simulink model "Quaternions"  (R2021b)
settings: Solver=VariableStepAuto  StartTime=0.0  StopTime=SimTime  MaxStep=1e-2  RelTol=1e-13
values from neighbouring files (symbols this model uses):
  q0 = [0 0 1 0]    [Lab_4.m]
libraries: robotcorelib x1, vrlib x1
settings Model: Creator=adity  LastModifiedBy=adity
settings SolverCC: AlgebraicLoopSolver=TrustRegion
settings DebuggingCC: SFMachineParentedDataDiag=warning

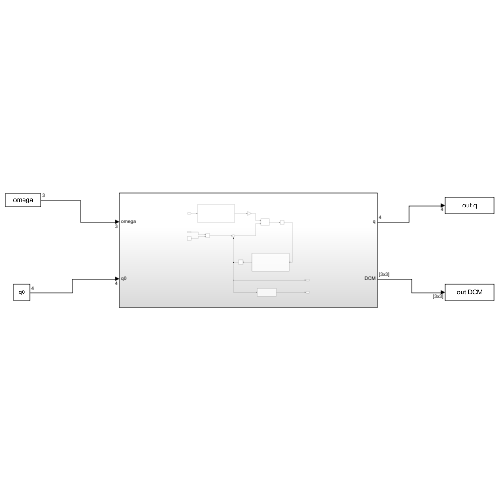
[thumbnail: Simulink's stored preview of the top-level diagram]
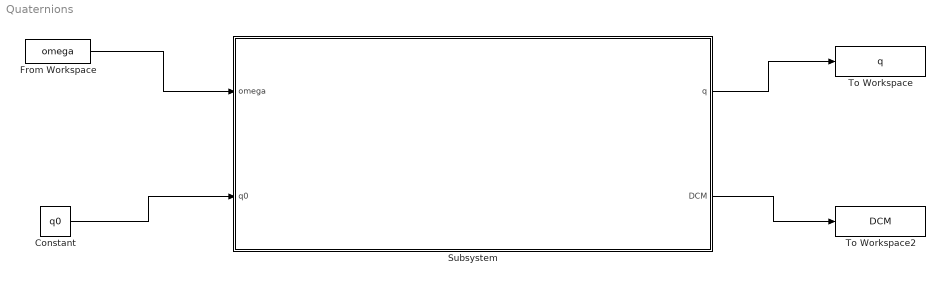
== system Quaternions ==
  Constant : Constant  Value=q0
  From Workspace : FromWorkspace  VariableName=omega
  Subsystem : Subsystem
  To Workspace : ToWorkspace  VariableName=q  SaveFormat=Timeseries  SampleTime=-1
  To Workspace2 : ToWorkspace  VariableName=DCM  SaveFormat=Timeseries  SampleTime=-1
  wires:
  From Workspace/1 -> Subsystem/1(omega)
  Constant/1 -> Subsystem/2(q0)
  Subsystem/1(q) -> To Workspace/1
  Subsystem/2(DCM) -> To Workspace2/1

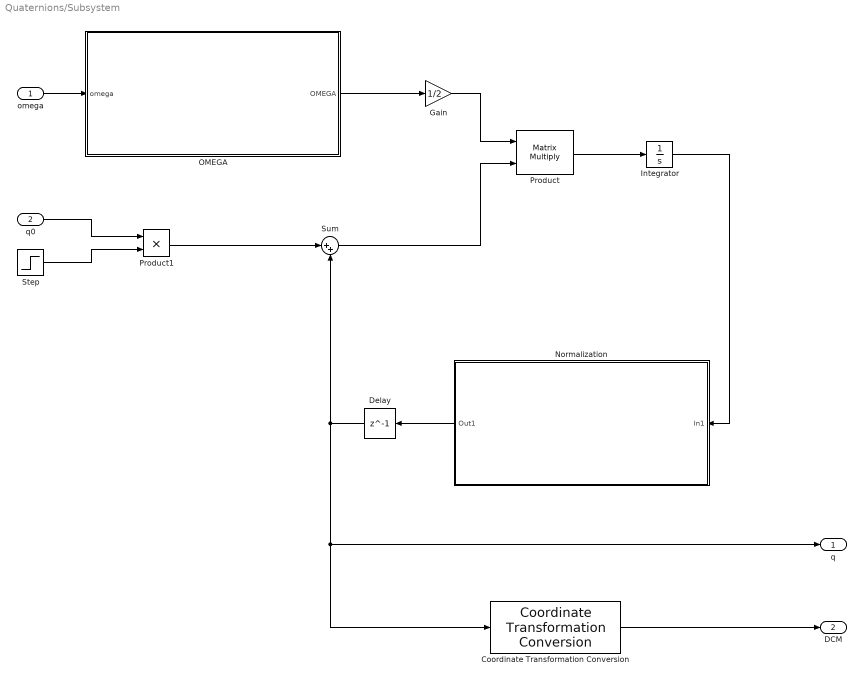
== system Quaternions/Subsystem ==
  omega : Inport
  q0 : Inport  Port=2
  Coordinate Transformation Conversion : robotcorelib/Coordinate Transformation Conversion  InputRepresentation=Quaternion  InputEulerSequence=ZYX  ShowTrVecInputPort=on  OutputRepresentation=Rotation Matrix  OutputEulerSequence=ZYX  ShowTrVecOutputPort=on  SimulateUsing=Interpreted execution
      settings: SourceProductBaseCode=NV,RO,RR,UV
  Delay : Delay  DelayLength=1
  Gain : Gain  Gain=1/2
  Integrator : Integrator  InitialCondition=q0
  Normalization : Subsystem
  OMEGA : Subsystem
  Product : Product  Multiplication=Matrix(*)
  Product1 : Product
  Step : Step  Time=0.01  Before=1  After=0  SampleTime=0
  Sum : Sum  Inputs=|++
  q : Outport
  DCM : Outport  Port=2
  wires:
  OMEGA/1(OMEGA) -> Gain/1
  Gain/1 -> Product/1
  Product/1 -> Integrator/1
  q0/1 -> Product1/1
  Step/1 -> Product1/2
  Product1/1 -> Sum/1
  Sum/1 -> Product/2
  Integrator/1 -> Normalization/1(In1)
  omega/1 -> OMEGA/1(omega)
  Normalization/1(Out1) -> Delay/1
  Delay/1 -> Coordinate Transformation Conversion/1, q/1, Sum/2
  Coordinate Transformation Conversion/1 -> DCM/1

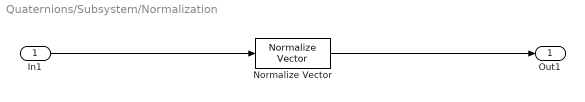
== system Quaternions/Subsystem/Normalization ==
  In1 : Inport
  Normalize Vector : vrlib/Utilities/Normalize Vector  maxzero=0
  Out1 : Outport
  wires:
  In1/1 -> Normalize Vector/1
  Normalize Vector/1 -> Out1/1

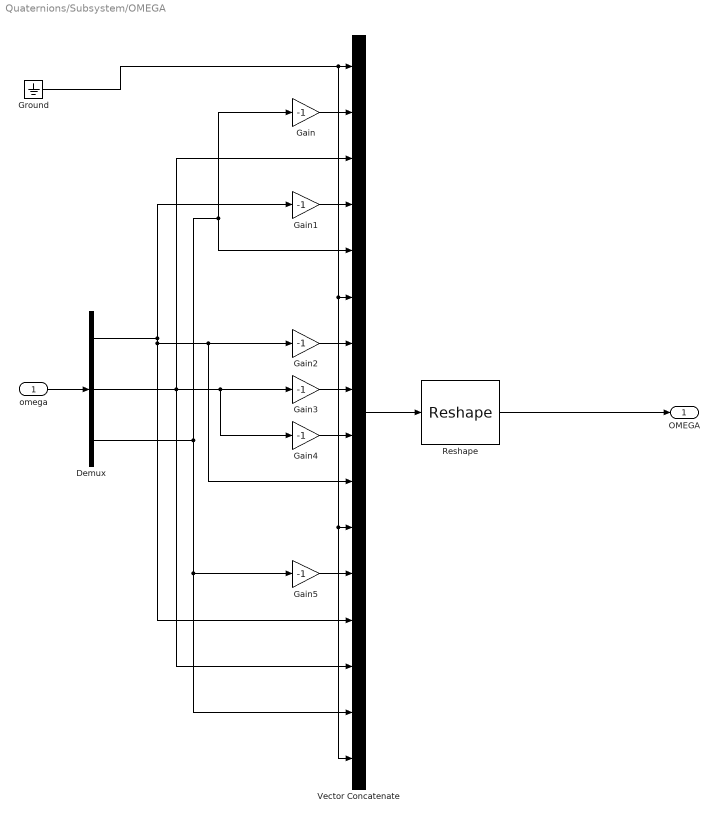
== system Quaternions/Subsystem/OMEGA ==
  omega : Inport
  Demux : Demux  Outputs=3
  Gain{,1..5} (6 alike) : Gain  Gain=-1
  Ground : Ground
  Reshape : Reshape  OutputDimensionality=Customize  OutputDimensions=[4,4]
  Vector Concatenate : Concatenate  NumInputs=16
  OMEGA : Outport
  wires:
  omega/1 -> Demux/1
  Vector Concatenate/1 -> Reshape/1
  Reshape/1 -> OMEGA/1
  Ground/1 -> Vector Concatenate/16, Vector Concatenate/11, Vector Concatenate/6, Vector Concatenate/1
  Gain/1 -> Vector Concatenate/2
  Demux/3 -> Gain5/1, Vector Concatenate/15, Gain/1, Vector Concatenate/5
  Demux/2 -> Gain3/1, Gain4/1, Vector Concatenate/3, Vector Concatenate/14
  Gain1/1 -> Vector Concatenate/4
  Demux/1 -> Gain2/1, Vector Concatenate/10, Vector Concatenate/13, Gain1/1
  Gain2/1 -> Vector Concatenate/7
  Gain3/1 -> Vector Concatenate/8
  Gain4/1 -> Vector Concatenate/9
  Gain5/1 -> Vector Concatenate/12
